simulink model "video"  (Simulink 7.7)
settings: Solver=ode45  StartTime=0.0  StopTime=10.0  RelTol=1e-3
undefined symbols (not defined in the file or in its folder): gray, M, N, Rec, SDTV, sz
libraries: vipmisc x23, dspsigops x7, dspobslib x6, viptransforms x6, viputilities x6, vipsnks x3, vipconversions x3, vipobslib x1, dspsrcs4 x1
(part 1 of 2)
settings Model: Creator=katsikas  LastModifiedBy=katsikas

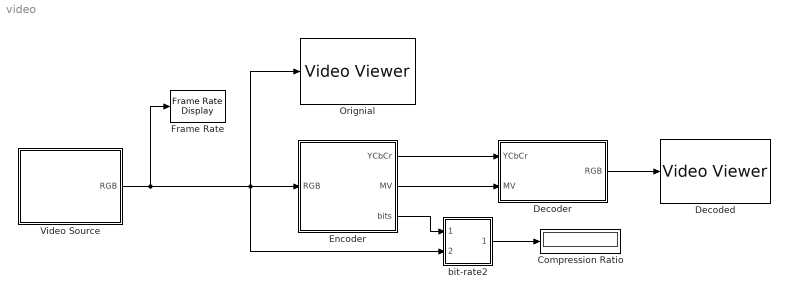
== system video ==
  Compression Ratio : Display
  Decoded : vipsnks/Video Viewer  inputType=Obsolete7b  imagePorts=One multidimensional signal  useColorMap=off  colormapValue=gray(256)  specRange=off  minInputVal=0  maxInputVal=255  FigPos=[801 443 175 140]  AxisZoom=on  trueSizedOnce=on  OpenAtMdlStart=on
  Decoder : Subsystem
  Encoder : Subsystem
  Frame Rate : vipsnks/Frame Rate Display  UpdateRate=10
  Orignial : vipsnks/Video Viewer  inputType=Obsolete7b  imagePorts=One multidimensional signal  useColorMap=off  colormapValue=gray(256)  specRange=off  minInputVal=0  maxInputVal=255  FigPos=[800 270 170 136]  AxisZoom=on  trueSizedOnce=on  OpenAtMdlStart=on
  Video Source : Subsystem
  bit-rate2 : Subsystem
  wires:
  Encoder/2(MV) -> Decoder/2(MV)
  Encoder/3(bits) -> bit-rate2/1(bits)
  bit-rate2/1(ratio) -> Compression Ratio/1
  Decoder/1(RGB) -> Decoded/1
  Encoder/1(YCbCr) -> Decoder/1(YCbCr)
  Video Source/1(RGB) -> Frame Rate/1, Encoder/1(RGB), Orignial/1, bit-rate2/2(RGB)

== system video/Decoder ==
  YCbCr : Inport
  MV : Inport  Port=2
  Block Processing : Subsystem  DialogController=vipDDGCreate  DialogControllerArgs=DataTag1  TreatAsAtomicUnit=on  mask(Block Processing){NumI=7, ParamPort=on, NumO=3, Blocksize={[20 1], [20 1], [20 1], [46 46],[23 23], [23 23], [1 2]}, Overlapsize={[0 0],[0 0],[0 0], [30 30], [15 15], [15 15],[0 0]}, Traverse=Row-wise}
      mask prompts: NumI "Number of inputs:"; ParamPort "Add port to supply subsystem parameters"; NumO "Number of outputs:"; Blocksize "Block size:"; Overlapsize "Overlap size:"; Traverse "Order of traversing:"
      mask help:
      | Repeats a user-specified operation on submatrices of the input matrix.
      |
      | This block extracts submatrices of a user-specified size from the input matrix. It sends each submatrix to a subsystem for processing, and then reassembles each subsystem output into the output matrix.
      |
      | Use the Block size and Overlap parameters to specify the size and overlap of each submatrix in cell array format.
      mask init:
      | errmsg = vipblkblockproc(gcbh, NumI, NumO, Blocksize, Overlapsize, Traverse, ParamPort);
      | error(errmsg);
      settings: CopyFcn=set_param(gcb,'LinkStatus','none');
      mask Help: eval('helpview(fullfile(docroot,''toolbox'',''vision'',''vision.map''),''vipblockprocessing'')');
      mask StyleString: edit,checkbox,edit,edit,edit,popup(Row-wise|Column-wise)
      mask Display:
      | disp('Block\n Processing');
      | 
      | if ((NumI == 1) && ParamPort)
      |     port_label('input', 1, 'I');
      | end
      | 
      | if (NumI > 1)
      |     for (i = 1:NumI)
      |         port_label('input', i, ['I' int2str(i)]);
      |     end
      | end
      | 
      | if (ParamPort)
      |     port_label('input', NumI+1, 'P');
      | end
  Chroma Resampling : vipconversions/Chroma Resampling  resampling=4:2:0 (MPEG2) to 4:4:4  interpolation=linear  antialiasing=Default  hcoeff=[0.2 0.6 0.2]  vcoeff=[0.5 0.5]  isInputTransposed=off
  Color Space  Conversion : vipconversions/Color Space  Conversion  conversion=Obsolete  conversionActive=Y'CbCr to R'G'B'  wp_str=D65  rec=Rec. 601 (SDTV)  sys=1125/60/2:1  imagePorts=One multidimensional signal
  Delay and pad : Subsystem
  Split 3-D into  separate 2-D signals : Subsystem
  Vector Concatenate1 : Concatenate  NumInputs=3  Mode=Multidimensional array  ConcatenateDimension=3
  RGB : Outport
  wires:
  Color Space  Conversion/1 -> RGB/1
  Block Processing/1(Out) -> Delay and pad/1(In1), Vector Concatenate1/1
  Block Processing/3(Out3) -> Delay and pad/3(In3), Chroma Resampling/2
  Block Processing/2(Out2) -> Delay and pad/2(In2), Chroma Resampling/1
  Delay and pad/1(Out1) -> Block Processing/4(In4)
  Delay and pad/2(Out2) -> Block Processing/5(In5)
  Delay and pad/3(Out3) -> Block Processing/6(In6)
  MV/1 -> Block Processing/7(In7)
  [IP] -> Block Processing/8(P)
  Vector Concatenate1/1 -> Color Space  Conversion/1
  Chroma Resampling/1 -> Vector Concatenate1/2
  Chroma Resampling/2 -> Vector Concatenate1/3
  YCbCr/1 -> Split 3-D into  separate 2-D signals/1(Image)
  Split 3-D into  separate 2-D signals/1(Y) -> Block Processing/1(In)
  Split 3-D into  separate 2-D signals/2(Cb) -> Block Processing/2(In2)
  Split 3-D into  separate 2-D signals/3(Cr) -> Block Processing/3(In3)

== system video/Encoder ==
  RGB : Inport
  Block Processing : Subsystem  DialogController=vipDDGCreate  DialogControllerArgs=DataTag5  TreatAsAtomicUnit=on  mask(Block Processing){NumI=6, ParamPort=on, NumO=5, Blocksize={[16 16],[8 8],[8 8],[46 46],[23 23],[23 23]}, Overlapsize={[0 0],[0 0],[0 0],[30 30],[15 15],[15 15]}, Traverse=Row-wise}
      mask prompts: NumI "Number of inputs:"; ParamPort "Add port to supply subsystem parameters"; NumO "Number of outputs:"; Blocksize "Block size:"; Overlapsize "Overlap size:"; Traverse "Order of traversing:"
      mask help:
      | Repeats a user-specified operation on submatrices of the input matrix.
      |
      | This block extracts submatrices of a user-specified size from the input matrix. It sends each submatrix to a subsystem for processing, and then reassembles each subsystem output into the output matrix.
      |
      | Use the Block size and Overlap parameters to specify the size and overlap of each submatrix in cell array format.
      mask init:
      | errmsg = vipblkblockproc(gcbh, NumI, NumO, Blocksize, Overlapsize, Traverse, ParamPort);
      | error(errmsg);
      settings: CopyFcn=set_param(gcb,'LinkStatus','none');
      mask Help: eval('helpview(fullfile(docroot,''toolbox'',''vision'',''vision.map''),''vipblockprocessing'')');
      mask StyleString: edit,checkbox,edit,edit,edit,popup(Row-wise|Column-wise)
      mask Display:
      | disp('Block\n Processing');
      | 
      | if ((NumI == 1) && ParamPort)
      |     port_label('input', 1, 'I');
      | end
      | 
      | if (NumI > 1)
      |     for (i = 1:NumI)
      |         port_label('input', i, ['I' int2str(i)]);
      |     end
      | end
      | 
      | if (ParamPort)
      |     port_label('input', NumI+1, 'P');
      | end
  Chroma Resampling : vipconversions/Chroma Resampling  resampling=4:4:4 to 4:2:0 (MPEG2)  interpolation=linear  antialiasing=Default  hcoeff=[0.2 0.6 0.2]  vcoeff=[0.5 0.5]  isInputTransposed=off
  Delay and pad : Subsystem
  Splitter : Subsystem
  Vector Concatenate1 : Concatenate  NumInputs=3  Mode=Multidimensional array  ConcatenateDimension=3
  YCbCr : Outport
  MV : Outport  Port=2
  bits : Outport  Port=3
  wires:
  Delay and pad/1(Out1) -> Block Processing/4(In4)
  Delay and pad/2(Out2) -> Block Processing/5(In5)
  Delay and pad/3(Out3) -> Block Processing/6(In6)
  Block Processing/4(Out4) -> MV/1
  Chroma Resampling/1 -> Delay and pad/2(In2), Block Processing/2(In2)
  Chroma Resampling/2 -> Delay and pad/3(In3), Block Processing/3(In3)
  [IP] -> Block Processing/7(P)
  Block Processing/5(Out5) -> bits/1
  RGB/1 -> Splitter/1(Image)
  Splitter/1(Y) -> Delay and pad/1(In1), Block Processing/1(In)
  Splitter/2(Cb) -> Chroma Resampling/1
  Splitter/3(Cr) -> Chroma Resampling/2
  Block Processing/1(Out) -> Vector Concatenate1/1
  Block Processing/2(Out2) -> Vector Concatenate1/2
  Block Processing/3(Out3) -> Vector Concatenate1/3
  Vector Concatenate1/1 -> YCbCr/1

== system video/Video Source ==
  From Multimedia File : dspsrcs4/From Multimedia File  inputFilename=vipmen.avi  loop=on  numPlays=inf  outputStreams=Video only  videoDataType=single  audioDataType=int16  inheritSampleTime=on  userDefinedSampleTime=1/30  noAudioOutput=off  isIntensityVideo=off  fourcc=RGB  colorVideoFormat=One multidimensional signal  outputEOF=off  dataOrg=Column-major  audioFrameSize=1024  computeAudioFrameSize=off
  RGB : Outport
  wires:
  From Multimedia File/1 -> RGB/1

== system video/bit-rate2 ==
  bits : Inport
  RGB : Inport  Port=2
  Gain : Gain  Gain=24
  Matrix Sum : dspobslib/Matrix Sum  Dim=Columns  roundingMode=Floor  overflowMode=off
  Matrix Sum1 : dspobslib/Matrix Sum  Dim=Rows  roundingMode=Floor  overflowMode=off
  Product2 : Product  Inputs=*/  RndMeth=Zero
  Splitter -Y : Selector  NumberOfDimensions=3  IndexOptions=Select all,Select all,Index vector (dialog)  Indices=[],[],[1]  OutputSizes=1
  Width : Width
  ratio : Outport
  wires:
  Gain/1 -> Product2/1
  Width/1 -> Gain/1
  Matrix Sum1/1 -> Product2/2
  bits/1 -> Matrix Sum/1
  Matrix Sum/1 -> Matrix Sum1/1
  RGB/1 -> Splitter -Y/1
  Product2/1 -> ratio/1
  Splitter -Y/1 -> Width/1

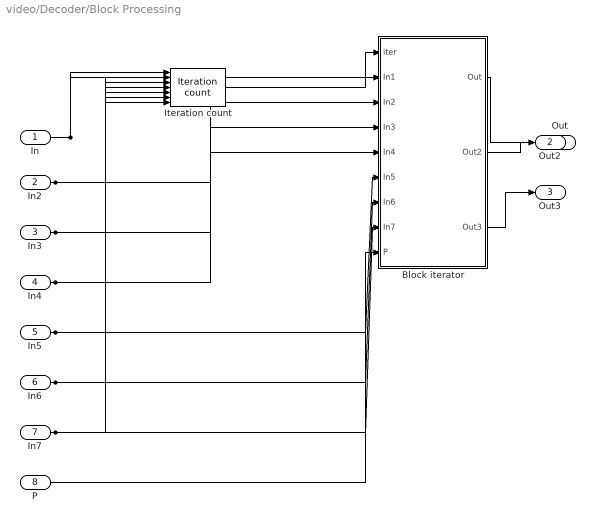
== system video/Decoder/Block Processing ==
  In : Inport
  In2 : Inport  Port=2
  In3 : Inport  Port=3
  In4 : Inport  Port=4
  In5 : Inport  Port=5
  In6 : Inport  Port=6
  In7 : Inport  Port=7
  P : Inport  Port=8
  Block iterator : Subsystem
      settings: CopyFcn=set_param(gcb,'ReferenceBlock','');
  Iteration count : vipmisc/Iteration count  NumI=NumI  blksize=Blocksize  ovlpsize=Overlapsize
  Out : Outport
  Out2 : Outport  Port=2
  Out3 : Outport  Port=3
  wires:
  Iteration count/1 -> Block iterator/1(iter)
  In/1 -> Iteration count/1, Block iterator/2(In1)
  Block iterator/1(Out) -> Out/1
  In2/1 -> Block iterator/3(In2), Iteration count/2
  In3/1 -> Block iterator/4(In3), Iteration count/3
  In4/1 -> Block iterator/5(In4), Iteration count/4
  In5/1 -> Block iterator/6(In5), Iteration count/5
  In6/1 -> Block iterator/7(In6), Iteration count/6
  In7/1 -> Block iterator/8(In7), Iteration count/7
  Block iterator/2(Out2) -> Out2/1
  Block iterator/3(Out3) -> Out3/1
  P/1 -> Block iterator/9(P)

== system video/Decoder/Delay and pad ==
  In1 : Inport
  In2 : Inport  Port=2
  In3 : Inport  Port=3
  2-D Pad : viputilities/Image Pad  method=Constant  valSrc=Specify via dialog  value=0  spec=Pad size  rowDirection=Both left and right  outRowsMode=User-specified  rowSize=15  outColSize=10  colDirection=Both top and bottom  outColsMode=User-specified  colSize=15  outRowSize=12  trunc_flag=None
  2-D Pad1 : viputilities/Image Pad  method=Constant  valSrc=Specify via dialog  value=0  spec=Pad size  rowDirection=Both left and right  outRowsMode=User-specified  rowSize=8  outColSize=10  colDirection=Both top and bottom  outColsMode=User-specified  colSize=8  outRowSize=12  trunc_flag=None
  2-D Pad2 : viputilities/Image Pad  method=Constant  valSrc=Specify via dialog  value=0  spec=Pad size  rowDirection=Both left and right  outRowsMode=User-specified  rowSize=8  outColSize=10  colDirection=Both top and bottom  outColsMode=User-specified  colSize=8  outRowSize=12  trunc_flag=None
  Delay : dspsigops/Delay  InputProcessing=Inherited (this choice will be removed - see release notes)  dly_unit=Samples  delay=1  ic_detail=off  dif_ic_for_ch=off  dif_ic_for_dly=off  ic=0  reset_popup=None
  Delay1 : dspsigops/Delay  InputProcessing=Inherited (this choice will be removed - see release notes)  dly_unit=Samples  delay=1  ic_detail=off  dif_ic_for_ch=off  dif_ic_for_dly=off  ic=0  reset_popup=None
  Delay2 : dspsigops/Delay  InputProcessing=Inherited (this choice will be removed - see release notes)  dly_unit=Samples  delay=1  ic_detail=off  dif_ic_for_ch=off  dif_ic_for_dly=off  ic=0  reset_popup=None
  Out1 : Outport
  Out2 : Outport  Port=2
  Out3 : Outport  Port=3
  wires:
  Delay/1 -> 2-D Pad/1
  In1/1 -> Delay/1
  2-D Pad/1 -> Out1/1
  Delay1/1 -> 2-D Pad1/1
  Delay2/1 -> 2-D Pad2/1
  In2/1 -> Delay1/1
  In3/1 -> Delay2/1
  2-D Pad1/1 -> Out2/1
  2-D Pad2/1 -> Out3/1

== system video/Decoder/Split 3-D into  separate 2-D signals ==
  Image : Inport
  Splitter -Cb : Selector  NumberOfDimensions=3  IndexOptions=Select all,Select all,Index vector (dialog)  Indices=[],[],[2]  OutputSizes=1
  Splitter -Cr : Selector  NumberOfDimensions=3  IndexOptions=Select all,Select all,Index vector (dialog)  Indices=[],[],[3]  OutputSizes=1
  Splitter -Y : Selector  NumberOfDimensions=3  IndexOptions=Select all,Select all,Index vector (dialog)  Indices=[],[],[1]  OutputSizes=1
  Y : Outport
  Cb : Outport  Port=2
  Cr : Outport  Port=3
  wires:
  Image/1 -> Splitter -Cb/1, Splitter -Cr/1, Splitter -Y/1
  Splitter -Y/1 -> Y/1
  Splitter -Cb/1 -> Cb/1
  Splitter -Cr/1 -> Cr/1

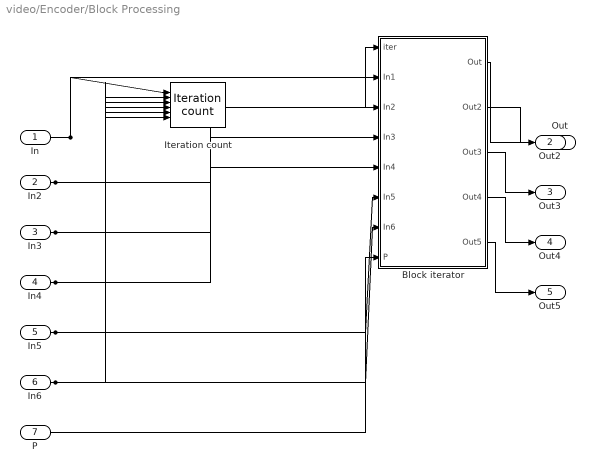
== system video/Encoder/Block Processing ==
  In : Inport
  In2 : Inport  Port=2
  In3 : Inport  Port=3
  In4 : Inport  Port=4
  In5 : Inport  Port=5
  In6 : Inport  Port=6
  P : Inport  Port=7
  Block iterator : Subsystem
      settings: CopyFcn=set_param(gcb,'ReferenceBlock','');
  Iteration count : vipmisc/Iteration count  NumI=NumI  blksize=Blocksize  ovlpsize=Overlapsize
  Out : Outport
  Out2 : Outport  Port=2
  Out3 : Outport  Port=3
  Out4 : Outport  Port=4
  Out5 : Outport  Port=5
  wires:
  Iteration count/1 -> Block iterator/1(iter)
  In/1 -> Iteration count/1, Block iterator/2(In1)
  Block iterator/1(Out) -> Out/1
  In2/1 -> Block iterator/3(In2), Iteration count/2
  In3/1 -> Block iterator/4(In3), Iteration count/3
  In4/1 -> Block iterator/5(In4), Iteration count/4
  In5/1 -> Block iterator/6(In5), Iteration count/5
  In6/1 -> Block iterator/7(In6), Iteration count/6
  Block iterator/2(Out2) -> Out2/1
  Block iterator/3(Out3) -> Out3/1
  Block iterator/4(Out4) -> Out4/1
  Block iterator/5(Out5) -> Out5/1
  P/1 -> Block iterator/8(P)

== system video/Encoder/Delay and pad ==
  In1 : Inport
  In2 : Inport  Port=2
  In3 : Inport  Port=3
  2-D Pad : viputilities/Image Pad  method=Constant  valSrc=Specify via dialog  value=0  spec=Pad size  rowDirection=Both left and right  outRowsMode=User-specified  rowSize=15  outColSize=10  colDirection=Both top and bottom  outColsMode=User-specified  colSize=15  outRowSize=12  trunc_flag=None
  2-D Pad1 : viputilities/Image Pad  method=Constant  valSrc=Specify via dialog  value=0  spec=Pad size  rowDirection=Both left and right  outRowsMode=User-specified  rowSize=8  outColSize=10  colDirection=Both top and bottom  outColsMode=User-specified  colSize=8  outRowSize=12  trunc_flag=None
  2-D Pad2 : viputilities/Image Pad  method=Constant  valSrc=Specify via dialog  value=0  spec=Pad size  rowDirection=Both left and right  outRowsMode=User-specified  rowSize=8  outColSize=10  colDirection=Both top and bottom  outColsMode=User-specified  colSize=8  outRowSize=12  trunc_flag=None
  Delay : dspsigops/Delay  InputProcessing=Inherited (this choice will be removed - see release notes)  dly_unit=Samples  delay=1  ic_detail=off  dif_ic_for_ch=off  dif_ic_for_dly=off  ic=0  reset_popup=None
  Delay1 : dspsigops/Delay  InputProcessing=Inherited (this choice will be removed - see release notes)  dly_unit=Samples  delay=1  ic_detail=off  dif_ic_for_ch=off  dif_ic_for_dly=off  ic=0  reset_popup=None
  Delay2 : dspsigops/Delay  InputProcessing=Inherited (this choice will be removed - see release notes)  dly_unit=Samples  delay=1  ic_detail=off  dif_ic_for_ch=off  dif_ic_for_dly=off  ic=0  reset_popup=None
  Out1 : Outport
  Out2 : Outport  Port=2
  Out3 : Outport  Port=3
  wires:
  In1/1 -> Delay/1
  Delay/1 -> 2-D Pad/1
  2-D Pad/1 -> Out1/1
  Delay1/1 -> 2-D Pad1/1
  Delay2/1 -> 2-D Pad2/1
  In2/1 -> Delay1/1
  2-D Pad1/1 -> Out2/1
  2-D Pad2/1 -> Out3/1
  In3/1 -> Delay2/1

== system video/Encoder/Splitter ==
  Image : Inport
  Splitter -Cb : Selector  NumberOfDimensions=3  IndexOptions=Select all,Select all,Index vector (dialog)  Indices=[],[],[2]  OutputSizes=1
  Splitter -Cr : Selector  NumberOfDimensions=3  IndexOptions=Select all,Select all,Index vector (dialog)  Indices=[],[],[3]  OutputSizes=1
  Splitter -Y : Selector  NumberOfDimensions=3  IndexOptions=Select all,Select all,Index vector (dialog)  Indices=[],[],[1]  OutputSizes=1
  Y : Outport
  Cb : Outport  Port=2
  Cr : Outport  Port=3
  wires:
  Splitter -Cr/1 -> Cr/1
  Splitter -Cb/1 -> Cb/1
  Splitter -Y/1 -> Y/1
  Image/1 -> Splitter -Y/1, Splitter -Cr/1, Splitter -Cb/1

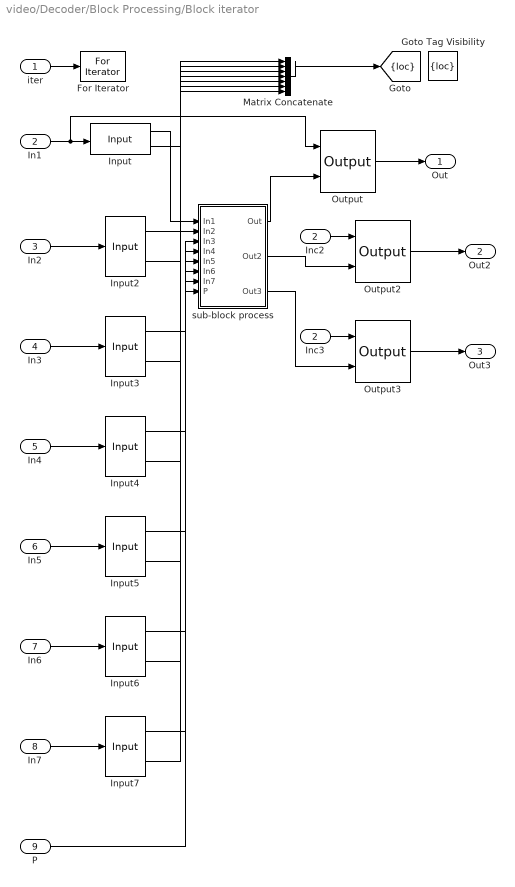
== system video/Decoder/Block Processing/Block iterator ==
  iter : Inport
  In1 : Inport  Port=2
  In2 : Inport  Port=3
  In3 : Inport  Port=4
  In4 : Inport  Port=5
  In5 : Inport  Port=6
  In6 : Inport  Port=7
  In7 : Inport  Port=8
  P : Inport  Port=9
  For Iterator : ForIterator  IterationSource=external  IterationLimit=(sz(1)/M)*(sz(2)/N)  ShowIterationPort=off  IndexMode=Zero-based  IterationVariableDataType=double
  Goto Tag Visibility : GotoTagVisibility  GotoTag=loc
  Inc2 : InportShadow  Port=2
  Inc3 : InportShadow  Port=2
  Input : vipmisc/Input  SystemSampleTime=-1  Blocksize=Blocksize{1}  Overlapsize=Overlapsize{1}  tverse=Row-wise
  Input2 : vipmisc/Input  SystemSampleTime=-1  Blocksize=Blocksize{2}  Overlapsize=Overlapsize{2}  tverse=Row-wise
  Input3 : vipmisc/Input  SystemSampleTime=-1  Blocksize=Blocksize{3}  Overlapsize=Overlapsize{3}  tverse=Row-wise
  Input4 : vipmisc/Input  SystemSampleTime=-1  Blocksize=Blocksize{4}  Overlapsize=Overlapsize{4}  tverse=Row-wise
  Input5 : vipmisc/Input  SystemSampleTime=-1  Blocksize=Blocksize{5}  Overlapsize=Overlapsize{5}  tverse=Row-wise
  Input6 : vipmisc/Input  SystemSampleTime=-1  Blocksize=Blocksize{6}  Overlapsize=Overlapsize{6}  tverse=Row-wise
  Input7 : vipmisc/Input  SystemSampleTime=-1  Blocksize=Blocksize{7}  Overlapsize=Overlapsize{7}  tverse=Row-wise
  Matrix Concatenate : Concatenate  NumInputs=7  Mode=Multidimensional array  ConcatenateDimension=2
  Output : vipmisc/Output  SystemSampleTime=-1  Blocksize=Blocksize{1}  Overlapsize=Overlapsize{1}  tverse=Row-wise
  Output2 : vipmisc/Output  SystemSampleTime=-1  Blocksize=Blocksize{1}  Overlapsize=Overlapsize{1}  tverse=Row-wise
  Output3 : vipmisc/Output  SystemSampleTime=-1  Blocksize=Blocksize{1}  Overlapsize=Overlapsize{1}  tverse=Row-wise
  sub-block process : Subsystem
  Out : Outport
  Out2 : Outport  Port=2
  Out3 : Outport  Port=3
  tag scope: loc=scoped
  wires:
  Matrix Concatenate/1 -> [loc]
  Input/2 -> Matrix Concatenate/1
  Input/1 -> sub-block process/1(In1)
  iter/1 -> For Iterator/1
  In1/1 -> Input/1, Output/1
  Output/1 -> Out/1
  sub-block process/1(Out) -> Output/2
  Input2/2 -> Matrix Concatenate/2
  In2/1 -> Input2/1
  Input2/1 -> sub-block process/2(In2)
  Input3/2 -> Matrix Concatenate/3
  In3/1 -> Input3/1
  Input3/1 -> sub-block process/3(In3)
  Input4/2 -> Matrix Concatenate/4
  In4/1 -> Input4/1
  Input4/1 -> sub-block process/4(In4)
  Input5/2 -> Matrix Concatenate/5
  In5/1 -> Input5/1
  Input5/1 -> sub-block process/5(In5)
  Input6/2 -> Matrix Concatenate/6
  In6/1 -> Input6/1
  Input6/1 -> sub-block process/6(In6)
  Input7/2 -> Matrix Concatenate/7
  In7/1 -> Input7/1
  Input7/1 -> sub-block process/7(In7)
  Inc2/1 -> Output2/1
  Output2/1 -> Out2/1
  sub-block process/2(Out2) -> Output2/2
  Inc3/1 -> Output3/1
  Output3/1 -> Out3/1
  sub-block process/3(Out3) -> Output3/2
  P/1 -> sub-block process/8(P)

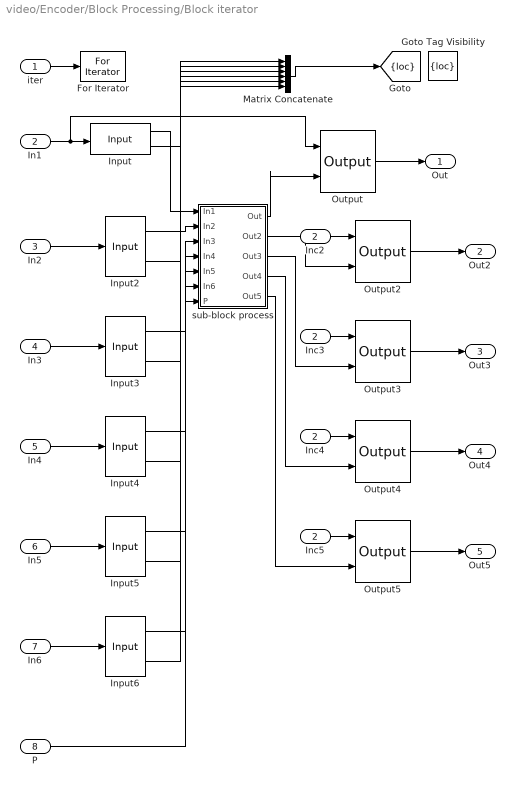
== system video/Encoder/Block Processing/Block iterator ==
  iter : Inport
  In1 : Inport  Port=2
  In2 : Inport  Port=3
  In3 : Inport  Port=4
  In4 : Inport  Port=5
  In5 : Inport  Port=6
  In6 : Inport  Port=7
  P : Inport  Port=8
  For Iterator : ForIterator  IterationSource=external  IterationLimit=(sz(1)/M)*(sz(2)/N)  ShowIterationPort=off  IndexMode=Zero-based  IterationVariableDataType=double
  Goto Tag Visibility : GotoTagVisibility  GotoTag=loc
  Inc{2..5} (4 alike) : InportShadow  Port=2
  Input : vipmisc/Input  SystemSampleTime=-1  Blocksize=Blocksize{1}  Overlapsize=Overlapsize{1}  tverse=Row-wise
  Input2 : vipmisc/Input  SystemSampleTime=-1  Blocksize=Blocksize{2}  Overlapsize=Overlapsize{2}  tverse=Row-wise
  Input3 : vipmisc/Input  SystemSampleTime=-1  Blocksize=Blocksize{3}  Overlapsize=Overlapsize{3}  tverse=Row-wise
  Input4 : vipmisc/Input  SystemSampleTime=-1  Blocksize=Blocksize{4}  Overlapsize=Overlapsize{4}  tverse=Row-wise
  Input5 : vipmisc/Input  SystemSampleTime=-1  Blocksize=Blocksize{5}  Overlapsize=Overlapsize{5}  tverse=Row-wise
  Input6 : vipmisc/Input  SystemSampleTime=-1  Blocksize=Blocksize{6}  Overlapsize=Overlapsize{6}  tverse=Row-wise
  Matrix Concatenate : Concatenate  NumInputs=6  Mode=Multidimensional array  ConcatenateDimension=2
  Output{,2..5} (5 alike) : vipmisc/Output  SystemSampleTime=-1  Blocksize=Blocksize{1}  Overlapsize=Overlapsize{1}  tverse=Row-wise
  sub-block process : Subsystem
  Out : Outport
  Out2 : Outport  Port=2
  Out3 : Outport  Port=3
  Out4 : Outport  Port=4
  Out5 : Outport  Port=5
  tag scope: loc=scoped
  wires:
  Matrix Concatenate/1 -> [loc]
  Input/2 -> Matrix Concatenate/1
  Input/1 -> sub-block process/1(In1)
  iter/1 -> For Iterator/1
  In1/1 -> Input/1, Output/1
  Output/1 -> Out/1
  sub-block process/1(Out) -> Output/2
  Input2/2 -> Matrix Concatenate/2
  In2/1 -> Input2/1
  Input2/1 -> sub-block process/2(In2)
  Input3/2 -> Matrix Concatenate/3
  In3/1 -> Input3/1
  Input3/1 -> sub-block process/3(In3)
  Input4/2 -> Matrix Concatenate/4
  In4/1 -> Input4/1
  Input4/1 -> sub-block process/4(In4)
  Input5/2 -> Matrix Concatenate/5
  In5/1 -> Input5/1
  Input5/1 -> sub-block process/5(In5)
  Input6/2 -> Matrix Concatenate/6
  In6/1 -> Input6/1
  Input6/1 -> sub-block process/6(In6)
  Inc2/1 -> Output2/1
  Output2/1 -> Out2/1
  sub-block process/2(Out2) -> Output2/2
  Inc3/1 -> Output3/1
  Output3/1 -> Out3/1
  sub-block process/3(Out3) -> Output3/2
  Inc4/1 -> Output4/1
  Output4/1 -> Out4/1
  sub-block process/4(Out4) -> Output4/2
  Inc5/1 -> Output5/1
  Output5/1 -> Out5/1
  sub-block process/5(Out5) -> Output5/2
  P/1 -> sub-block process/7(P)

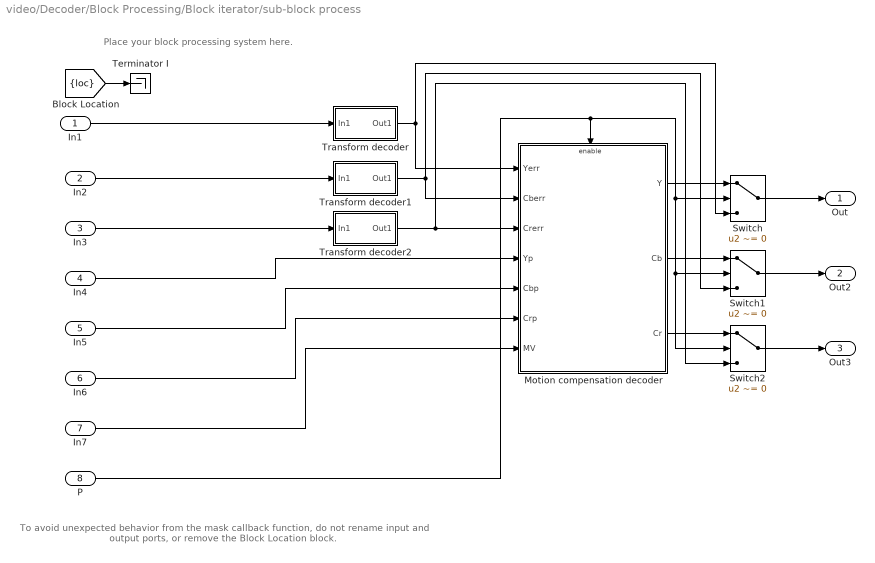
== system video/Decoder/Block Processing/Block iterator/sub-block process ==
  note: To avoid unexpected behavior from the mask
      | callback function, do not rename input and output ports,
      | or remove the Block Location block.
  note: Place your block
      | processing system here.
  In1 : Inport
  In2 : Inport  Port=2
  In3 : Inport  Port=3
  In4 : Inport  Port=4
  In5 : Inport  Port=5
  In6 : Inport  Port=6
  In7 : Inport  Port=7
  P : Inport  Port=8
  Motion compensation decoder : Subsystem
  Switch : Switch  Criteria=u2 ~= 0
  Switch1 : Switch  Criteria=u2 ~= 0
  Switch2 : Switch  Criteria=u2 ~= 0
  Terminator I : Terminator
  Transform decoder : Subsystem
  Transform decoder1 : Subsystem
  Transform decoder2 : Subsystem
  Out : Outport
  Out2 : Outport  Port=2
  Out3 : Outport  Port=3
  wires:
  [loc] -> Terminator I/1
  P/1 -> Motion compensation decoder/Enable, Switch/2, Switch1/2, Switch2/2
  In1/1 -> Transform decoder/1(In1)
  In2/1 -> Transform decoder1/1(In1)
  In3/1 -> Transform decoder2/1(In1)
  Transform decoder/1(Out1) -> Motion compensation decoder/1(Yerr), Switch/3
  Transform decoder1/1(Out1) -> Motion compensation decoder/2(Cberr), Switch1/3
  Transform decoder2/1(Out1) -> Motion compensation decoder/3(Crerr), Switch2/3
  In4/1 -> Motion compensation decoder/4(Yp)
  In5/1 -> Motion compensation decoder/5(Cbp)
  In6/1 -> Motion compensation decoder/6(Crp)
  In7/1 -> Motion compensation decoder/7(MV)
  Motion compensation decoder/1(Y) -> Switch/1
  Motion compensation decoder/2(Cb) -> Switch1/1
  Motion compensation decoder/3(Cr) -> Switch2/1
  Switch/1 -> Out/1
  Switch1/1 -> Out2/1
  Switch2/1 -> Out3/1

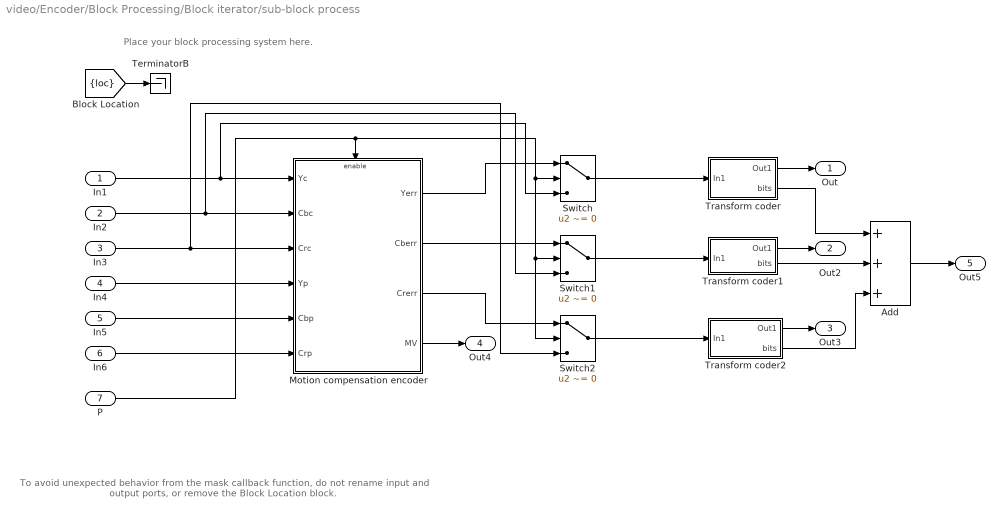
== system video/Encoder/Block Processing/Block iterator/sub-block process ==
  note: To avoid unexpected behavior from the mask
      | callback function, do not rename input and output ports,
      | or remove the Block Location block.
  note: Place your block
      | processing system here.
  In1 : Inport
  In2 : Inport  Port=2
  In3 : Inport  Port=3
  In4 : Inport  Port=4
  In5 : Inport  Port=5
  In6 : Inport  Port=6
  P : Inport  Port=7
  Add : Sum  Inputs=+++
  Motion compensation encoder : Subsystem
  Switch : Switch  Criteria=u2 ~= 0
  Switch1 : Switch  Criteria=u2 ~= 0
  Switch2 : Switch  Criteria=u2 ~= 0
  TerminatorB : Terminator
  Transform coder : Subsystem
  Transform coder1 : Subsystem
  Transform coder2 : Subsystem
  Out : Outport
  Out2 : Outport  Port=2
  Out3 : Outport  Port=3
  Out4 : Outport  Port=4
  Out5 : Outport  Port=5
  wires:
  [loc] -> TerminatorB/1
  P/1 -> Motion compensation encoder/Enable, Switch/2, Switch1/2, Switch2/2
  In1/1 -> Motion compensation encoder/1(Yc), Switch/3
  In2/1 -> Motion compensation encoder/2(Cbc), Switch1/3
  In3/1 -> Motion compensation encoder/3(Crc), Switch2/3
  In4/1 -> Motion compensation encoder/4(Yp)
  In5/1 -> Motion compensation encoder/5(Cbp)
  In6/1 -> Motion compensation encoder/6(Crp)
  Motion compensation encoder/1(Yerr) -> Switch/1
  Motion compensation encoder/2(Cberr) -> Switch1/1
  Motion compensation encoder/3(Crerr) -> Switch2/1
  Switch/1 -> Transform coder/1(In1)
  Switch1/1 -> Transform coder1/1(In1)
  Switch2/1 -> Transform coder2/1(In1)
  Transform coder/1(Out1) -> Out/1
  Transform coder/2(bits) -> Add/1
  Transform coder1/2(bits) -> Add/2
  Transform coder2/1(Out1) -> Out3/1
  Transform coder2/2(bits) -> Add/3
  Add/1 -> Out5/1
  Transform coder1/1(Out1) -> Out2/1
  Motion compensation encoder/4(MV) -> Out4/1

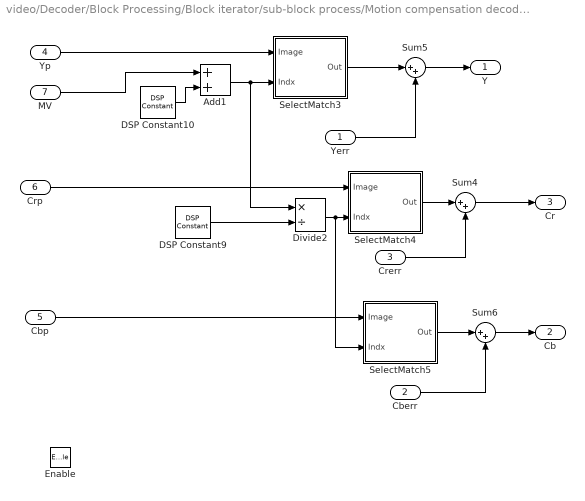
== system video/Decoder/Block Processing/Block iterator/sub-block process/Motion compensation decoder ==
  Yerr : Inport
  Cberr : Inport  Port=2
  Crerr : Inport  Port=3
  Yp : Inport  Port=4
  Cbp : Inport  Port=5
  Crp : Inport  Port=6
  MV : Inport  Port=7
  Enable : EnablePort  PropagateVarSize=During execution
  Add1 : Sum  OutDataTypeStr=single
  DSP Constant10 : dspobslib/DSP Constant  SystemSampleTime=-1  Value=15  SampleMode=Discrete  discreteOutput=Sample-based  continuousOutput=Sample-based  sampTime=-1  framePeriod=2  dataType=int32  isSigned=on  wordLen=16  udDataType=sfix(16)  fracBitsMode=Best precision  numFracBits=15  InterpretAs1D=-inf  Ts=-inf  FramebasedOutput=-inf
      settings: additionalParams=on  allowOverrides=off
  DSP Constant9 : dspobslib/DSP Constant  SystemSampleTime=-1  Value=2  SampleMode=Discrete  discreteOutput=Sample-based  continuousOutput=Sample-based  sampTime=-1  framePeriod=2  dataType=int32  isSigned=on  wordLen=16  udDataType=sfix(16)  fracBitsMode=Best precision  numFracBits=15  InterpretAs1D=-inf  Ts=-inf  FramebasedOutput=-inf
      settings: additionalParams=on  allowOverrides=off
  Divide2 : Product  Inputs=*/  OutDataTypeStr=int8  RndMeth=Zero
  SelectMatch3 : Subsystem
  SelectMatch4 : Subsystem
  SelectMatch5 : Subsystem
  Sum4 : Sum  Inputs=|++
  Sum5 : Sum  Inputs=|++
  Sum6 : Sum  Inputs=|++
  Y : Outport
  Cb : Outport  Port=2
  Cr : Outport  Port=3
  wires:
  Yerr/1 -> Sum5/2
  SelectMatch3/1(Out) -> Sum5/1
  DSP Constant10/1 -> Add1/2
  Add1/1 -> SelectMatch3/2(Indx), Divide2/1
  Sum5/1 -> Y/1
  Divide2/1 -> SelectMatch4/2(Indx), SelectMatch5/2(Indx)
  DSP Constant9/1 -> Divide2/2
  SelectMatch4/1(Out) -> Sum4/1
  Sum4/1 -> Cr/1
  SelectMatch5/1(Out) -> Sum6/1
  Crp/1 -> SelectMatch4/1(Image)
  Crerr/1 -> Sum4/2
  Cbp/1 -> SelectMatch5/1(Image)
  Cberr/1 -> Sum6/2
  Yp/1 -> SelectMatch3/1(Image)
  Sum6/1 -> Cb/1
  MV/1 -> Add1/1

== system video/Decoder/Block Processing/Block iterator/sub-block process/Transform decoder ==
  In1 : Inport
  2D IDCT : viptransforms/2-D IDCT  CompMethod=Table lookup  Dimension=0  TableOpt=Speed  BitRevOrder=off  SkipNorm=off  firstCoeffDataTypeStr=Inherit: Same word length as input  firstCoeffLastDataTypeStr=Inherit: Same word length as input  outputMin=[]  outputMax=[]  roundingMode=Floor  overflowMode=off
  AC zigzag1 : Selector  IndexOptions=Index vector (dialog)  Indices="[1     3     4    10    11    21    22    36     2     5     9    12    20    23    35    37     6     8    13    19    24    34    38    49     7    14    18    25    33    39    48    50    15    17    26    32    40    47    51     58    16    27    31    41    46    52    57    59    28    30    42    45     53    56    60    63    29    43    44    54    55    61    62    64]"  OutputSizes=1
  Bit Unpack : Stateflow chart  TreatAsAtomicUnit=on
  Gain1 : Gain  Gain=16/255
  Gain2 : Gain  Gain=16/255
  Matrix Concatenation : Concatenate  Mode=Multidimensional array
  Reshape1 : Reshape  OutputDimensionality=Customize  OutputDimensions=[8,8]
  Zero Pad : dspsigops/Pad  padAlong=Columns and rows  dimsToPad=1  valSrc=Specify via dialog  padVal=0  spec=Output size  padNumOutRowsSpecMethod=User-specified  numOutRows=16  padNumOutColsSpecMethod=User-specified  numOutCols=16  isVarDimsMode=off  padBeginning=0  padEnd=0  outSizeMode=User-specified  outSize=1  padSigAt=End  trunc_flag=None  roundingMode=Floor  overflowMode=off  truncOrWrapMode=Truncate  wrap_flag=None
  select 0 : Selector  IndexMode=Zero-based  IndexOptions=Index vector (dialog)  Indices=0  OutputSizes=8, 8
  select 1 : Selector  IndexMode=Zero-based  IndexOptions=Starting index (dialog)  Indices=1  OutputSizes=63
  Out1 : Outport
  wires:
  Gain2/1 -> Matrix Concatenation/2
  select 1/1 -> Gain2/1
  Gain1/1 -> Matrix Concatenation/1
  Matrix Concatenation/1 -> Reshape1/1
  select 0/1 -> Gain1/1
  AC zigzag1/1 -> select 1/1, select 0/1
  Bit Unpack/1(out) -> AC zigzag1/1
  2D IDCT/1 -> Out1/1
  Zero Pad/1 -> 2D IDCT/1
  Reshape1/1 -> Zero Pad/1
  In1/1 -> Bit Unpack/1(in)

== system video/Decoder/Block Processing/Block iterator/sub-block process/Transform decoder1 ==
  In1 : Inport
  2D IDCT : viptransforms/2-D IDCT  CompMethod=Table lookup  Dimension=0  TableOpt=Speed  BitRevOrder=off  SkipNorm=off  firstCoeffDataTypeStr=Inherit: Same word length as input  firstCoeffLastDataTypeStr=Inherit: Same word length as input  outputMin=[]  outputMax=[]  roundingMode=Floor  overflowMode=off
  AC zigzag1 : Selector  IndexOptions=Index vector (dialog)  Indices="[1     3     4    10    11    21    22    36     2     5     9    12    20    23    35    37     6     8    13    19    24    34    38    49     7    14    18    25    33    39    48    50    15    17    26    32    40    47    51     58    16    27    31    41    46    52    57    59    28    30    42    45     53    56    60    63    29    43    44    54    55    61    62    64]"  OutputSizes=1
  Bit Unpack : Stateflow chart  TreatAsAtomicUnit=on
  Gain1 : Gain  Gain=8/255
  Gain2 : Gain  Gain=8/255
  Matrix Concatenation : Concatenate  Mode=Multidimensional array
  Reshape1 : Reshape  OutputDimensionality=Customize  OutputDimensions=[8,8]
  select 0 : Selector  IndexMode=Zero-based  IndexOptions=Index vector (dialog)  Indices=0  OutputSizes=8, 8
  select 1 : Selector  IndexMode=Zero-based  IndexOptions=Starting index (dialog)  Indices=1  OutputSizes=63
  Out1 : Outport
  wires:
  In1/1 -> Bit Unpack/1(in)
  Reshape1/1 -> 2D IDCT/1
  2D IDCT/1 -> Out1/1
  AC zigzag1/1 -> select 0/1, select 1/1
  select 0/1 -> Gain1/1
  Matrix Concatenation/1 -> Reshape1/1
  Gain1/1 -> Matrix Concatenation/1
  select 1/1 -> Gain2/1
  Gain2/1 -> Matrix Concatenation/2
  Bit Unpack/1(out) -> AC zigzag1/1

== system video/Decoder/Block Processing/Block iterator/sub-block process/Transform decoder2 ==
  In1 : Inport
  2D IDCT : viptransforms/2-D IDCT  CompMethod=Table lookup  Dimension=0  TableOpt=Speed  BitRevOrder=off  SkipNorm=off  firstCoeffDataTypeStr=Inherit: Same word length as input  firstCoeffLastDataTypeStr=Inherit: Same word length as input  outputMin=[]  outputMax=[]  roundingMode=Floor  overflowMode=off
  AC zigzag1 : Selector  IndexOptions=Index vector (dialog)  Indices="[1     3     4    10    11    21    22    36     2     5     9    12    20    23    35    37     6     8    13    19    24    34    38    49     7    14    18    25    33    39    48    50    15    17    26    32    40    47    51     58    16    27    31    41    46    52    57    59    28    30    42    45     53    56    60    63    29    43    44    54    55    61    62    64]"  OutputSizes=1
  Bit Unpack : Stateflow chart  TreatAsAtomicUnit=on
  Gain1 : Gain  Gain=8/255
  Gain2 : Gain  Gain=8/255
  Matrix Concatenation : Concatenate  Mode=Multidimensional array
  Reshape1 : Reshape  OutputDimensionality=Customize  OutputDimensions=[8,8]
  select 0 : Selector  IndexMode=Zero-based  IndexOptions=Index vector (dialog)  Indices=(0)  OutputSizes=8,8
  select 1 : Selector  IndexMode=Zero-based  IndexOptions=Starting index (dialog)  Indices=(1)  OutputSizes=63
  Out1 : Outport
  wires:
  Gain2/1 -> Matrix Concatenation/2
  select 1/1 -> Gain2/1
  Gain1/1 -> Matrix Concatenation/1
  Matrix Concatenation/1 -> Reshape1/1
  select 0/1 -> Gain1/1
  AC zigzag1/1 -> select 1/1, select 0/1
  2D IDCT/1 -> Out1/1
  Reshape1/1 -> 2D IDCT/1
  In1/1 -> Bit Unpack/1(in)
  Bit Unpack/1(out) -> AC zigzag1/1

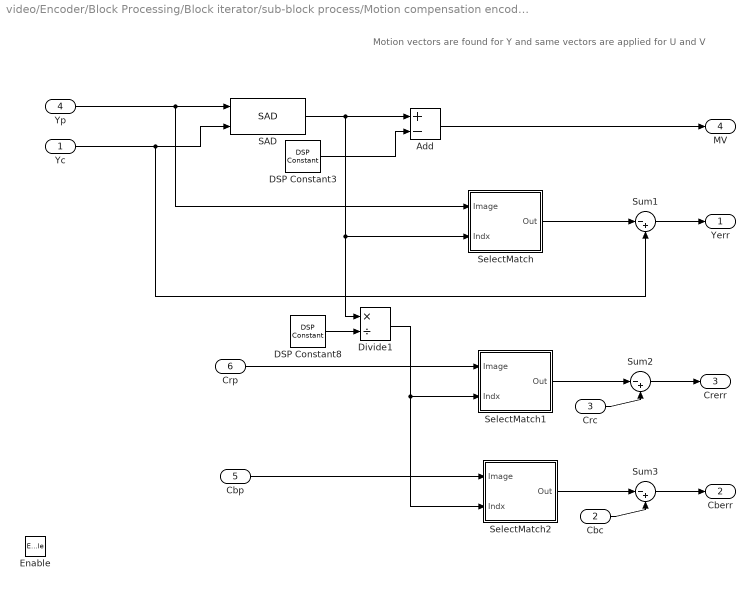
== system video/Encoder/Block Processing/Block iterator/sub-block process/Motion compensation encoder ==
  note: Motion vectors are found for Y and same
      |  vectors are applied for U and V
  Yc : Inport
  Cbc : Inport  Port=2
  Crc : Inport  Port=3
  Yp : Inport  Port=4
  Cbp : Inport  Port=5
  Crp : Inport  Port=6
  Enable : EnablePort  PropagateVarSize=During execution
  Add : Sum  Inputs=+-
  DSP Constant3 : dspobslib/DSP Constant  SystemSampleTime=-1  Value=15  SampleMode=Discrete  discreteOutput=Sample-based  continuousOutput=Sample-based  sampTime=-1  framePeriod=2  dataType=Inherit via back propagation  isSigned=on  wordLen=16  udDataType=sfix(16)  fracBitsMode=Best precision  numFracBits=15  InterpretAs1D=-inf  Ts=-inf  FramebasedOutput=-inf
      settings: additionalParams=on  allowOverrides=off
  DSP Constant8 : dspobslib/DSP Constant  SystemSampleTime=-1  Value=2  SampleMode=Discrete  discreteOutput=Sample-based  continuousOutput=Sample-based  sampTime=-1  framePeriod=2  dataType=Inherit via back propagation  isSigned=on  wordLen=16  udDataType=sfix(16)  fracBitsMode=Best precision  numFracBits=15  InterpretAs1D=-inf  Ts=-inf  FramebasedOutput=-inf
      settings: additionalParams=on  allowOverrides=off
  Divide1 : Product  Inputs=*/  OutDataTypeStr=int8  RndMeth=Zero
  SAD : vipobslib/SAD  output=Minimum SAD value index  method=Three-step  roi=off  invalidROI=Ignore  nearbyPel=off  nearbySize=3  roundingMode=Floor  overflowMode=off
  SelectMatch : Subsystem
  SelectMatch1 : Subsystem
  SelectMatch2 : Subsystem
  Sum1 : Sum  Inputs=|-+  OutDataTypeStr=Inherit: Same as first input
  Sum2 : Sum  Inputs=|-+  OutDataTypeStr=Inherit: Same as first input
  Sum3 : Sum  Inputs=|-+  OutDataTypeStr=Inherit: Same as first input
  Yerr : Outport
  Cberr : Outport  Port=2
  Crerr : Outport  Port=3
  MV : Outport  Port=4
  wires:
  Yp/1 -> SAD/1, SelectMatch/1(Image)
  Yc/1 -> Sum1/2, SAD/2
  DSP Constant3/1 -> Add/2
  Add/1 -> MV/1
  SelectMatch/1(Out) -> Sum1/1
  Sum1/1 -> Yerr/1
  DSP Constant8/1 -> Divide1/2
  Divide1/1 -> SelectMatch1/2(Indx), SelectMatch2/2(Indx)
  SelectMatch1/1(Out) -> Sum2/1
  Crc/1 -> Sum2/2
  Sum2/1 -> Crerr/1
  Crp/1 -> SelectMatch1/1(Image)
  Cbp/1 -> SelectMatch2/1(Image)
  SelectMatch2/1(Out) -> Sum3/1
  Cbc/1 -> Sum3/2
  Sum3/1 -> Cberr/1
  SAD/1 -> Add/1, SelectMatch/2(Indx), Divide1/1

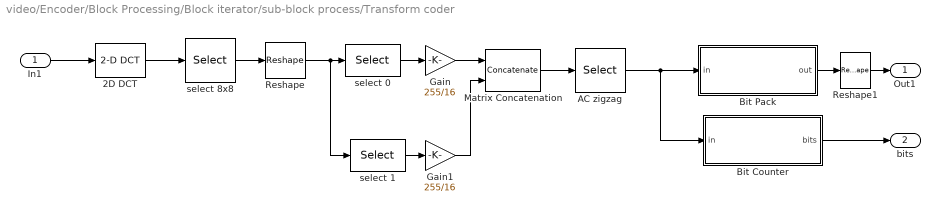
== system video/Encoder/Block Processing/Block iterator/sub-block process/Transform coder ==
  In1 : Inport
  2D DCT : viptransforms/2-D DCT  CompMethod=Table lookup  Dimension=0  TableOpt=Speed  BitRevOrder=off  SkipNorm=off  firstCoeffDataTypeStr=Inherit: Same word length as input  firstCoeffLastDataTypeStr=Inherit: Same word length as input  outputMin=[]  outputMax=[]  roundingMode=Floor  overflowMode=off
  AC zigzag : Selector  IndexOptions=Index vector (dialog)  Indices="([0  8     1     2     9    16    24    17    10     3     4    11    18    25  32    40    33    26    19    12     5     6    13    20    27    34    41  48    56    49    42    35    28    21    14     7    15    22    29    36  43    50    57    58    51    44    37    30    23    31    38    45    52  59    60    53    46    39    47    54    61    62    55    63]+1)"  OutputSizes=1
  Bit Counter : Stateflow chart  TreatAsAtomicUnit=on
  Bit Pack : Stateflow chart  TreatAsAtomicUnit=on
  Gain : Gain  Gain=255/16
  Gain1 : Gain  Gain=255/16
  Matrix Concatenation : Concatenate  Mode=Multidimensional array
  Reshape : Reshape  OutputDimensionality=Column vector (2-D)  OutputDimensions=[8,8]
  Reshape1 : Reshape  OutputDimensionality=Column vector (2-D)  OutputDimensions=[8,8]
  select 0 : Selector  IndexMode=Zero-based  IndexOptions=Index vector (dialog)  Indices=(0)  OutputSizes=8,8
  select 1 : Selector  IndexMode=Zero-based  IndexOptions=Starting index (dialog)  Indices=(1)  OutputSizes=63
  select 8x8 : Selector  NumberOfDimensions=2  IndexMode=Zero-based  IndexOptions=Starting index (dialog),Starting index (dialog)  Indices=(0),(0)  OutputSizes=8,8
  Out1 : Outport
  bits : Outport  Port=2
  wires:
  Bit Counter/1(bits) -> bits/1
  Gain1/1 -> Matrix Concatenation/2
  select 1/1 -> Gain1/1
  Gain/1 -> Matrix Concatenation/1
  Matrix Concatenation/1 -> AC zigzag/1
  select 0/1 -> Gain/1
  Reshape/1 -> select 1/1, select 0/1
  Bit Pack/1(out) -> Reshape1/1
  Reshape1/1 -> Out1/1
  2D DCT/1 -> select 8x8/1
  In1/1 -> 2D DCT/1
  AC zigzag/1 -> Bit Counter/1(in), Bit Pack/1(in)
  select 8x8/1 -> Reshape/1

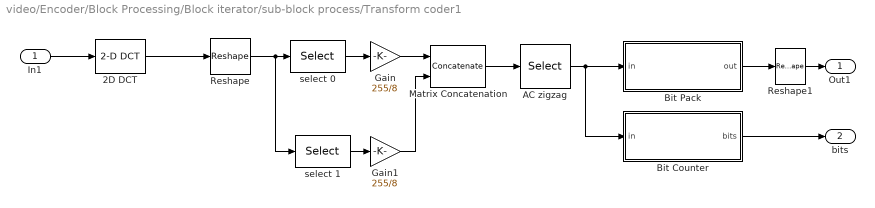
== system video/Encoder/Block Processing/Block iterator/sub-block process/Transform coder1 ==
  In1 : Inport
  2D DCT : viptransforms/2-D DCT  CompMethod=Table lookup  Dimension=0  TableOpt=Speed  BitRevOrder=off  SkipNorm=off  firstCoeffDataTypeStr=Inherit: Same word length as input  firstCoeffLastDataTypeStr=Inherit: Same word length as input  outputMin=[]  outputMax=[]  roundingMode=Floor  overflowMode=off
  AC zigzag : Selector  IndexOptions=Index vector (dialog)  Indices="([0  8     1     2     9    16    24    17    10     3     4    11    18    25  32    40    33    26    19    12     5     6    13    20    27    34    41  48    56    49    42    35    28    21    14     7    15    22    29    36  43    50    57    58    51    44    37    30    23    31    38    45    52  59    60    53    46    39    47    54    61    62    55    63]+1)"  OutputSizes=1
  Bit Counter : Stateflow chart  TreatAsAtomicUnit=on
  Bit Pack : Stateflow chart  TreatAsAtomicUnit=on
  Gain : Gain  Gain=255/8
  Gain1 : Gain  Gain=255/8
  Matrix Concatenation : Concatenate  Mode=Multidimensional array
  Reshape : Reshape  OutputDimensionality=Column vector (2-D)  OutputDimensions=[8,8]
  Reshape1 : Reshape  OutputDimensionality=Column vector (2-D)  OutputDimensions=[8,8]
  select 0 : Selector  IndexMode=Zero-based  IndexOptions=Index vector (dialog)  Indices=(0)  OutputSizes=8,8
  select 1 : Selector  IndexMode=Zero-based  IndexOptions=Starting index (dialog)  Indices=(1)  OutputSizes=63
  Out1 : Outport
  bits : Outport  Port=2
  wires:
  Bit Counter/1(bits) -> bits/1
  In1/1 -> 2D DCT/1
  2D DCT/1 -> Reshape/1
  Reshape1/1 -> Out1/1
  Reshape/1 -> select 0/1, select 1/1
  select 0/1 -> Gain/1
  Matrix Concatenation/1 -> AC zigzag/1
  Gain/1 -> Matrix Concatenation/1
  select 1/1 -> Gain1/1
  Gain1/1 -> Matrix Concatenation/2
  AC zigzag/1 -> Bit Counter/1(in), Bit Pack/1(in)
  Bit Pack/1(out) -> Reshape1/1

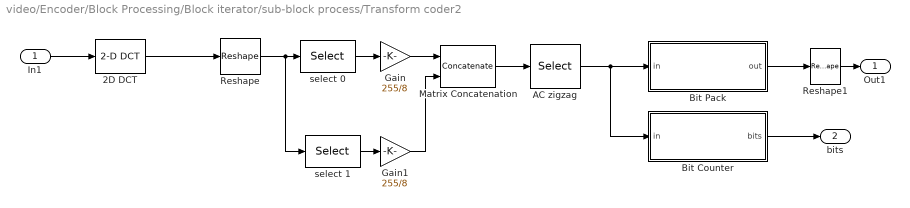
== system video/Encoder/Block Processing/Block iterator/sub-block process/Transform coder2 ==
  In1 : Inport
  2D DCT : viptransforms/2-D DCT  CompMethod=Table lookup  Dimension=0  TableOpt=Speed  BitRevOrder=off  SkipNorm=off  firstCoeffDataTypeStr=Inherit: Same word length as input  firstCoeffLastDataTypeStr=Inherit: Same word length as input  outputMin=[]  outputMax=[]  roundingMode=Floor  overflowMode=off
  AC zigzag : Selector  IndexOptions=Index vector (dialog)  Indices="([0  8     1     2     9    16    24    17    10     3     4    11    18    25  32    40    33    26    19    12     5     6    13    20    27    34    41  48    56    49    42    35    28    21    14     7    15    22    29    36  43    50    57    58    51    44    37    30    23    31    38    45    52  59    60    53    46    39    47    54    61    62    55    63]+1)"  OutputSizes=1
  Bit Counter : Stateflow chart  TreatAsAtomicUnit=on
  Bit Pack : Stateflow chart  TreatAsAtomicUnit=on
  Gain : Gain  Gain=255/8
  Gain1 : Gain  Gain=255/8
  Matrix Concatenation : Concatenate  Mode=Multidimensional array
  Reshape : Reshape  OutputDimensionality=Column vector (2-D)  OutputDimensions=[8,8]
  Reshape1 : Reshape  OutputDimensionality=Column vector (2-D)  OutputDimensions=[8,8]
  select 0 : Selector  IndexMode=Zero-based  IndexOptions=Index vector (dialog)  Indices=(0)  OutputSizes=8,8
  select 1 : Selector  IndexMode=Zero-based  IndexOptions=Starting index (dialog)  Indices=(1)  OutputSizes=63
  Out1 : Outport
  bits : Outport  Port=2
  wires:
  Bit Counter/1(bits) -> bits/1
  Gain1/1 -> Matrix Concatenation/2
  select 1/1 -> Gain1/1
  Gain/1 -> Matrix Concatenation/1
  Matrix Concatenation/1 -> AC zigzag/1
  select 0/1 -> Gain/1
  Reshape/1 -> select 1/1, select 0/1
  Reshape1/1 -> Out1/1
  2D DCT/1 -> Reshape/1
  In1/1 -> 2D DCT/1
  AC zigzag/1 -> Bit Counter/1(in), Bit Pack/1(in)
  Bit Pack/1(out) -> Reshape1/1

== system video/Decoder/Block Processing/Block iterator/sub-block process/Motion compensation decoder/SelectMatch3 ==
  Image : Inport
  Indx : Inport  Port=2
  Selector3 : Selector  NumberOfDimensions=2  IndexMode=Zero-based  InputPortWidth=3  IndexOptions=Starting index (port),Starting index (port)  Indices=1,1  OutputSizes=16, 16
  Selector4 : Selector  InputPortWidth=2  IndexOptions=Index vector (dialog)  Indices=1  OutputSizes=1
  Selector5 : Selector  InputPortWidth=2  IndexOptions=Index vector (dialog)  Indices=2  OutputSizes=1
  Out : Outport
  wires:
  Selector3/1 -> Out/1
  Indx/1 -> Selector5/1, Selector4/1
  Image/1 -> Selector3/1
  Selector5/1 -> Selector3/3
  Selector4/1 -> Selector3/2

== system video/Decoder/Block Processing/Block iterator/sub-block process/Motion compensation decoder/SelectMatch4 ==
  Image : Inport
  Indx : Inport  Port=2
  Selector3 : Selector  NumberOfDimensions=2  IndexMode=Zero-based  InputPortWidth=3  IndexOptions=Starting index (port),Starting index (port)  Indices=1,1  OutputSizes=8, 8
  Selector4 : Selector  InputPortWidth=2  IndexOptions=Index vector (dialog)  Indices=1  OutputSizes=1
  Selector5 : Selector  InputPortWidth=2  IndexOptions=Index vector (dialog)  Indices=2  OutputSizes=1
  Out : Outport
  wires:
  Selector4/1 -> Selector3/2
  Selector5/1 -> Selector3/3
  Image/1 -> Selector3/1
  Indx/1 -> Selector4/1, Selector5/1
  Selector3/1 -> Out/1

== system video/Decoder/Block Processing/Block iterator/sub-block process/Motion compensation decoder/SelectMatch5 ==
  Image : Inport
  Indx : Inport  Port=2
  Selector3 : Selector  NumberOfDimensions=2  IndexMode=Zero-based  InputPortWidth=3  IndexOptions=Starting index (port),Starting index (port)  Indices=1,1  OutputSizes=8, 8
  Selector4 : Selector  InputPortWidth=2  IndexOptions=Index vector (dialog)  Indices=1  OutputSizes=1
  Selector5 : Selector  InputPortWidth=2  IndexOptions=Index vector (dialog)  Indices=2  OutputSizes=1
  Out : Outport
  wires:
  Selector3/1 -> Out/1
  Indx/1 -> Selector5/1, Selector4/1
  Image/1 -> Selector3/1
  Selector5/1 -> Selector3/3
  Selector4/1 -> Selector3/2

== system video/Encoder/Block Processing/Block iterator/sub-block process/Motion compensation encoder/SelectMatch ==
  Image : Inport
  Indx : Inport  Port=2
  Selector3 : Selector  NumberOfDimensions=2  IndexMode=Zero-based  InputPortWidth=3  IndexOptions=Starting index (port),Starting index (port)  Indices=(1),(1)  OutputSizes=16,16
  Selector4 : Selector  InputPortWidth=2  IndexOptions=Index vector (dialog)  Indices=(1)  OutputSizes=1
  Selector5 : Selector  InputPortWidth=2  IndexOptions=Index vector (dialog)  Indices=(2)  OutputSizes=1
  Out : Outport
  wires:
  Selector4/1 -> Selector3/2
  Selector5/1 -> Selector3/3
  Image/1 -> Selector3/1
  Indx/1 -> Selector4/1, Selector5/1
  Selector3/1 -> Out/1

== system video/Encoder/Block Processing/Block iterator/sub-block process/Motion compensation encoder/SelectMatch1 ==
  Image : Inport
  Indx : Inport  Port=2
  Selector3 : Selector  NumberOfDimensions=2  IndexMode=Zero-based  InputPortWidth=3  IndexOptions=Starting index (port),Starting index (port)  Indices=(1),(1)  OutputSizes=8,8
  Selector4 : Selector  InputPortWidth=2  IndexOptions=Index vector (dialog)  Indices=(1)  OutputSizes=1
  Selector5 : Selector  InputPortWidth=2  IndexOptions=Index vector (dialog)  Indices=(2)  OutputSizes=1
  Out : Outport
  wires:
  Selector3/1 -> Out/1
  Indx/1 -> Selector5/1, Selector4/1
  Image/1 -> Selector3/1
  Selector5/1 -> Selector3/3
  Selector4/1 -> Selector3/2

== system video/Encoder/Block Processing/Block iterator/sub-block process/Motion compensation encoder/SelectMatch2 ==
  Image : Inport
  Indx : Inport  Port=2
  Selector3 : Selector  NumberOfDimensions=2  IndexMode=Zero-based  InputPortWidth=3  IndexOptions=Starting index (port),Starting index (port)  Indices=(1),(1)  OutputSizes=8,8
  Selector4 : Selector  InputPortWidth=2  IndexOptions=Index vector (dialog)  Indices=(1)  OutputSizes=1
  Selector5 : Selector  InputPortWidth=2  IndexOptions=Index vector (dialog)  Indices=(2)  OutputSizes=1
  Out : Outport
  wires:
  Selector4/1 -> Selector3/2
  Selector5/1 -> Selector3/3
  Image/1 -> Selector3/1
  Indx/1 -> Selector4/1, Selector5/1
  Selector3/1 -> Out/1

== matlab function Encoder/Block Processing/Block iterator/sub-block process/Transform coder/Bit Counter ==
  data: in input double; bits output double
function bits = bitcounter(in)
% This bitcounter assumes that the input signal will be 
% huffman encoded and counts bits based on this assumption. Note 
% however that the Bit Pack and Bit Unpack blocks only perform
% run length encoding.

numacbits = 0;
run = 0;

dclen = [2, 3, 3, 3, 3, 3, 4, 5, 6, 7, 8, 9];

if (in(1) < 0) 
    dcval = uint32(-in(1)); 
else
    dcval = uint32(in(1)); 
end

for i=0:11
    if (dcval == 0) 
        break; 
    end
    dcval = uint32(bitshift(dcval,-1));
end
numdcbits = dclen(i+1) + i;

aclen = [2,  2,  3,  4,  5,  7,  8, 10, 16, 16,...
    4,  5,  7,  9, 11, 16, 16, 16, 16, 16,...
    5,  8, 10, 12, 16, 16, 16, 16, 16, 16,...
    6,  9, 12, 16, 16, 16, 16, 16, 16, 16,...
    6, 10, 16, 16, 16, 16, 16, 16, 16, 16,...
    7, 11, 16, 16, 16, 16, 16, 16, 16, 16,...
    7, 12, 16, 16, 16, 16, 16, 16, 16, 16,...
    8, 12, 16, 16, 16, 16, 16, 16, 16, 16,...
    9, 15, 16, 16, 16, 16, 16, 16, 16, 16,...
    9, 16, 16, 16, 16, 16, 16, 16, 16, 16,...
    9, 16, 16, 16, 16, 16, 16, 16, 16, 16,...
    10, 16, 16, 16, 16, 16, 16, 16, 16, 16,...
    10, 16, 16, 16, 16, 16, 16, 16, 16, 16,...
    11, 16, 16, 16, 16, 16, 16, 16, 16, 16,...
    16, 16, 16, 16, 16, 16, 16, 16, 16, 16,...
    16, 16, 16, 16, 16, 16, 16, 16, 16, 16];



for i=1:63
    if (in(i+1) == 0)
        run = run+1;
        if (i < 63)
            continue;
        end
    end
    
    if (in(i+1) < 0) 
        acval = uint32(-in(i+1)); 
    else
        acval = uint32(in(i+1));
    end

    for j=0:31
        if (acval == 0) 
            break; 
        end

        acval = uint32(bitshift(acval,-1));
    end
    
    while (run > 15)
        run = run-15;
        numacbits = numacbits+11;
    end

    numacbits = numacbits + aclen(run*10 + j+1) + j;
    run = 0;
end

if (run > 0) 
    numacbits = numacbits+4; 
end
     
bits = single(numacbits+numdcbits);
